simulink model "planar_quad_animation"  (R2015a)
settings: Solver=ode45  StartTime=0.0  StopTime=200  RelTol=1e-3
InitFcn:
  |  planar_quad_param
undefined symbols (not defined in the file or in its folder): AP, drawPlanarQuad, out
libraries: simulink x1
settings Model: Creator=ecestudent  LastModifiedBy=ecestudent

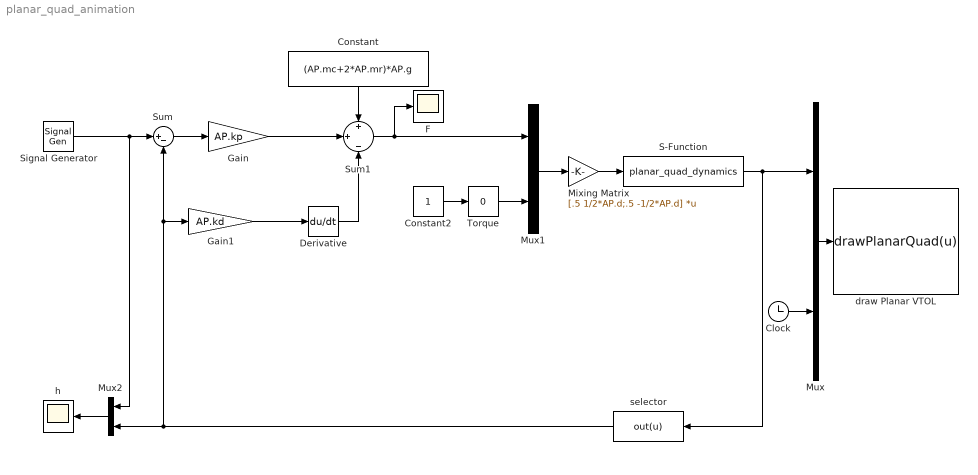
== system planar_quad_animation ==
  Clock : Clock
  Constant : Constant  Value=(AP.mc+2*AP.mr)*AP.g
  Constant2 : Constant
  Derivative : Derivative
  F : Scope
  Gain : Gain  Gain=AP.kp
  Gain1 : Gain  Gain=AP.kd
  Mixing Matrix : Gain  Gain=[.5 1/2*AP.d;.5 -1/2*AP.d]  Multiplication=Matrix(K*u)
  Mux : Mux  Inputs=2
  Mux1 : Mux  Inputs=2
  Mux2 : Mux  Inputs=2
  S-Function : S-Function  FunctionName=planar_quad_dynamics  Parameters=AP
  Signal Generator : SignalGenerator  WaveForm=square  Amplitude=2.5  Frequency=.02
  Sum : Sum  Inputs=|+-
  Sum1 : Sum  Inputs=+|+|-
  Torque : simulink/Math Operations/Slider Gain  low=-5  gain=0  high=5
  draw Planar VTOL : MATLABFcn  MATLABFcn=drawPlanarQuad(u)  OutputDimensions=0
      mask Display: image(imread('tv.jpg'))
  h : Scope
  selector : MATLABFcn  MATLABFcn=out(u)
  wires:
  Constant2/1 -> Torque/1
  Clock/1 -> Mux/2
  Mux/1 -> draw Planar VTOL/1
  Torque/1 -> Mux1/2
  S-Function/1 -> Mux/1, selector/1
  Sum/1 -> Gain/1
  Gain/1 -> Sum1/2
  Gain1/1 -> Derivative/1
  Derivative/1 -> Sum1/3
  Mux2/1 -> h/1
  Sum1/1 -> F/1, Mux1/1
  Constant/1 -> Sum1/1
  selector/1 -> Mux2/2, Gain1/1, Sum/2
  Mixing Matrix/1 -> S-Function/1
  Mux1/1 -> Mixing Matrix/1
  Signal Generator/1 -> Mux2/1, Sum/1
